simulink model "L3_T2_cascade_dq"  (R2026a)
settings: Solver=ode23tb  StartTime=0  StopTime=4  MaxStep=0.0005
settings Model: Creator=m  LastModifiedBy=m

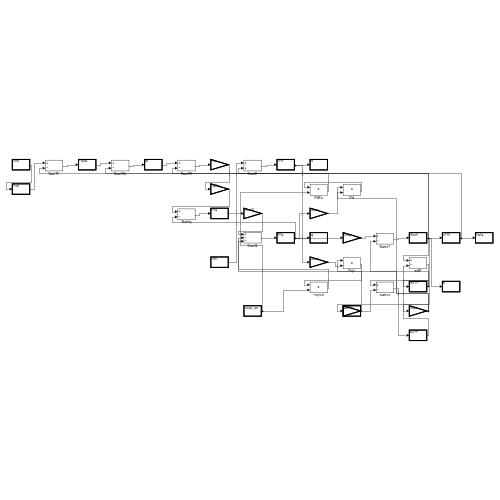
[thumbnail: Simulink's stored preview of the top-level diagram]
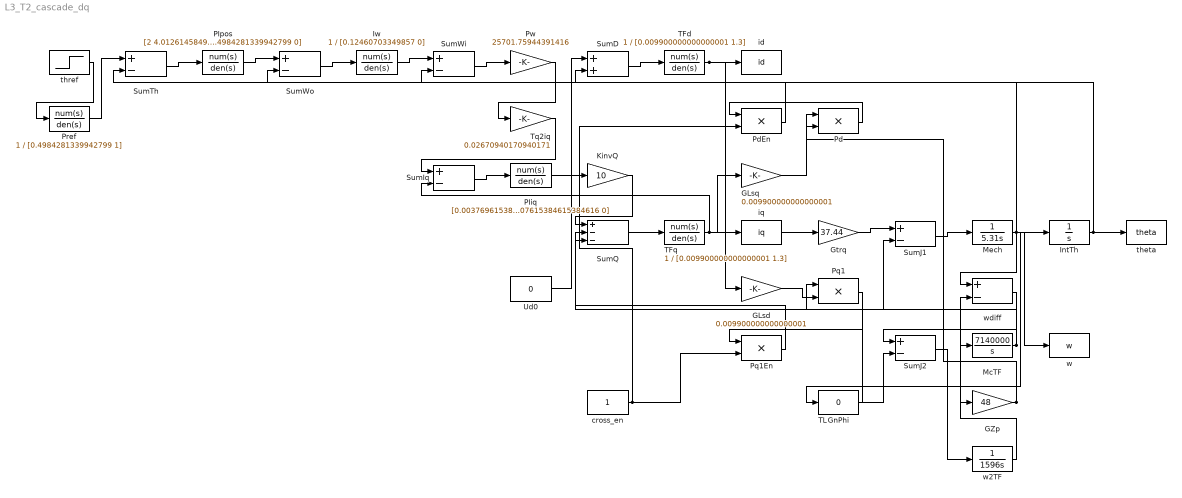
== system L3_T2_cascade_dq ==
  GLsd : Gain  Gain=0.009900000000000001
  GLsq : Gain  Gain=0.009900000000000001
  GZp : Gain  Gain=48
  GnPhi : Gain  Gain=0.52
  Gtrq : Gain  Gain=37.44
  IntTh : Integrator
  Iw : TransferFcn  Numerator=1  Denominator=[0.12460703349857 0]
  KinvQ : Gain  Gain=10
  McTF : TransferFcn  Numerator=7140000  Denominator=[1 0]
  Mech : TransferFcn  Numerator=1  Denominator=[5.31 0]
  PIiq : TransferFcn  Numerator=[0.003769615384615385 0.4950000000000001]  Denominator=[0.007615384615384616 0]
  PIpos : TransferFcn  Numerator=[2 4.012614584920185]  Denominator=[0.4984281339942799 0]
  Pd : Product
  PdEn : Product
  Pq1 : Product
  Pq1En : Product
  Pref : TransferFcn  Numerator=1  Denominator=[0.4984281339942799 1]
  Pw : Gain  Gain=25701.75944391416
  SumD : Sum
  SumIq : Sum  Inputs=+-
  SumJ1 : Sum  Inputs=+-
  SumJ2 : Sum  Inputs=+-
  SumQ : Sum  Inputs=+--
  SumTh : Sum  Inputs=+-
  SumWi : Sum  Inputs=+-
  SumWo : Sum  Inputs=+-
  TFd : TransferFcn  Numerator=1  Denominator=[0.009900000000000001 1.3]
  TFq : TransferFcn  Numerator=1  Denominator=[0.009900000000000001 1.3]
  TL : Constant  Value=0
  Tq2iq : Gain  Gain=0.02670940170940171
  Ud0 : Constant  Value=0
  cross_en : Constant
  id : ToWorkspace  VariableName=id  SaveFormat=Structure With Time  SampleTime=-1
  iq : ToWorkspace  VariableName=iq  SaveFormat=Structure With Time  SampleTime=-1
  theta : ToWorkspace  VariableName=theta  SaveFormat=Structure With Time  SampleTime=-1
  thref : Step  Time=0  FinalValue=0.08726646259971647  SampleTime=0
  w : ToWorkspace  VariableName=w  SaveFormat=Structure With Time  SampleTime=-1
  w2TF : TransferFcn  Numerator=1  Denominator=[1596 0]
  wdiff : Sum  Inputs=+-
  wires:
  SumD/1 -> TFd/1
  SumQ/1 -> TFq/1
  TFq/1 -> Gtrq/1, GLsq/1, SumIq/2, iq/1
  Gtrq/1 -> SumJ1/1
  SumJ1/1 -> Mech/1
  Mech/1 -> wdiff/1, GZp/1, IntTh/1, SumWi/2, SumWo/2, w/1
  w2TF/1 -> wdiff/2
  wdiff/1 -> McTF/1
  McTF/1 -> SumJ1/2, SumJ2/1
  SumJ2/1 -> w2TF/1
  GZp/1 -> Pd/1, Pq1/1, GnPhi/1
  GLsq/1 -> Pd/2
  Pd/1 -> PdEn/1
  cross_en/1 -> PdEn/2, Pq1En/2
  PdEn/1 -> SumD/2
  TFd/1 -> GLsd/1, id/1
  GLsd/1 -> Pq1/2
  Pq1/1 -> Pq1En/1
  Pq1En/1 -> SumQ/2
  GnPhi/1 -> SumQ/3
  thref/1 -> Pref/1
  Pref/1 -> SumTh/1
  SumTh/1 -> PIpos/1
  PIpos/1 -> SumWo/1
  SumWo/1 -> Iw/1
  Iw/1 -> SumWi/1
  SumWi/1 -> Pw/1
  Pw/1 -> Tq2iq/1
  Tq2iq/1 -> SumIq/1
  SumIq/1 -> PIiq/1
  PIiq/1 -> KinvQ/1
  KinvQ/1 -> SumQ/1
  Ud0/1 -> SumD/1
  TL/1 -> SumJ2/2
  IntTh/1 -> SumTh/2, theta/1
